simulink model "overall_simulator"  (R2018b)
settings: Solver=VariableStepAuto  StartTime=0.0  StopTime=100  RelTol=1e-3
InitFcn:
  | Iyy_lbft2= 261.096376; %last updated 7 Dec 2018
  | Iyy = 0.04214011 *Iyy_lbft2;
  | initial_conds
values from neighbouring files (symbols this model uses):
  desired_vel = 15    [initial_conds.m]
  flap_angle = 0    [initial_conds.m]
  initial_attitude = 0    [initial_conds.m]
  initial_incidence = 0    [initial_conds.m]
  motor_angle = 10    [initial_conds.m]
libraries: aerolibconvert2 x5, simulink x5, shared3dof x1, aerolibasang x1
settings Model: Creator=Devansh  LastModifiedBy=Alex
settings DebuggingCC: UnderSpecifiedDimensionMsg=warning
settings SFSimCC: SimUseLocalCustomCode=off
settings RTWCC: RTWUseLocalCustomCode=off
settings CodeAppCC: StateflowObjectComments=on

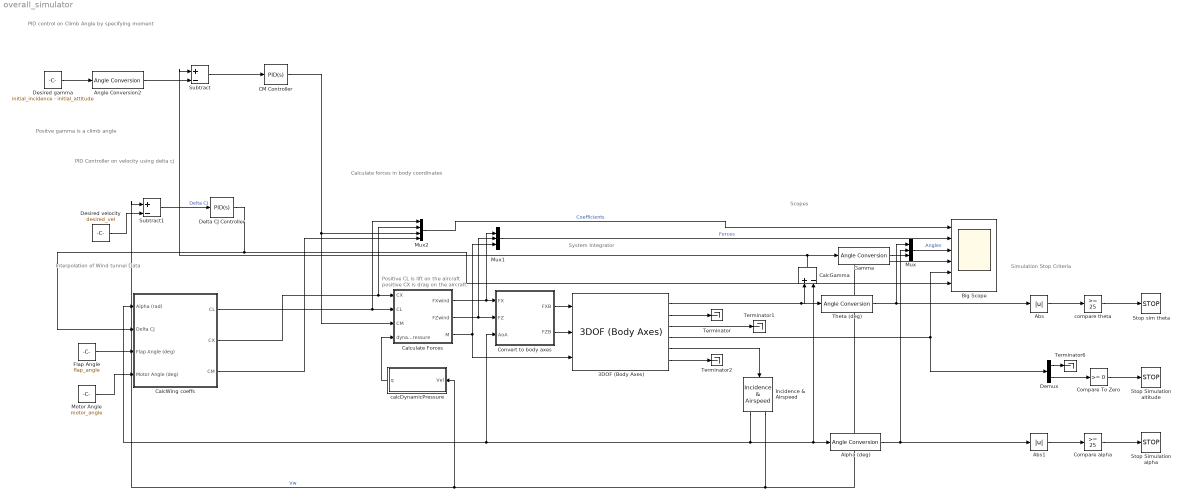
== system overall_simulator ==
  note: Positve gamma is a climb angle
  note: Scopes
  note: Simulation Stop Criteria
  note: System Integrator
  note: Calculate forces in body coordinates
  note: PID control on Climb Angle by specifying moment
  note: Interpolation of Wind tunnel Data
  note: PID Controller on velocity using delta cj
  note: Positive CL is lift on the aircraft
      | positive CX is drag on the aircraft
  3DOF (Body Axes) : shared3dof/3DOF (Body Axes)  units=Metric (MKS)  mtype=Fixed  v_ini=desired_vel  theta_ini=initial_attitude*pi/180  alpha_ini=initial_incidence*pi/180  pos_ini=initial_position  q_ini=0  mass=initial_mass  mass_e=0.5  mass_f=3.0  Iyy=Iyy  Iyy_e=0.5  Iyy_f=3.0  g_in=Internal  g=9.81  vre_flag=on  abi_flag=off  aMode=aMode  vel_statename=''  theta_statename=''  pos_statename=''  q_statename=''  mass_statename=''
      settings: SourceProductName=Aerospace Blockset  SourceProductBaseCode=AE
  Abs : Abs
  Abs1 : Abs
  Alpha (deg) : aerolibconvert2/Angle Conversion  IU=rad  OU=deg
  Angle Conversion2 : aerolibconvert2/Angle Conversion  IU=deg  OU=rad
  Big Scope : Scope  NumInputPorts=6
  CM Controller : simulink/Continuous/PID Controller  Controller=PID  Form=Parallel  TimeDomain=Continuous-time  SampleTime=-1  IntegratorMethod=Forward Euler  FilterMethod=Forward Euler  ControllerParametersSource=internal  P=-.005  I=0  D=-.05  UseFilter=on  N=100  TunerSelectOption=Frequency Response Based  InitialConditionSource=internal  InitialConditionForIntegrator=0  InitialConditionForFilter=0  DifferentiatorICPrevScaledInput=0  ExternalReset=none  TrackingMode=off  Kt=1  LimitOutput=off  UpperSaturationLimit=0.1  LowerSaturationLimit=-0.1  LinearizeAsGain=off  AntiWindupMode=none  Kb=1  POutMin=[]  POutMax=[]  IOutMin=[]  IOutMax=[]  DOutMin=[]  DOutMax=[]  NOutMin=[]  NOutMax=[]  SumOutMin=[]  SumOutMax=[]  SaturationOutMin=[]  SaturationOutMax=[]  PParamMin=[]  PParamMax=[]  IParamMin=[]  IParamMax=[]  DParamMin=[]  DParamMax=[]  NParamMin=[]  NParamMax=[]  KbParamMin=[]  KbParamMax=[]  KtParamMin=[]  KtParamMax=[]  KbOutMin=[]  KbOutMax=[]  KtOutMin=[]  KtOutMax=[]  IntegratorOutMin=[]  IntegratorOutMax=[]  FilterOutMin=[]  FilterOutMax=[]  SumI1OutMin=[]  SumI1OutMax=[]  SumI2OutMin=[]  SumI2OutMax=[]  SumI3OutMin=[]  SumI3OutMax=[]  SumI4OutMin=[]  SumI4OutMax=[]  SumDOutMin=[]  SumDOutMax=[]  DifferentiatorOutMin=[]  DifferentiatorOutMax=[]  FilterDiffOutCoefMin=[]  FilterDiffOutCoefMax=[]  ReciprocalOutMin=[]  ReciprocalOutMax=[]  SumDenOutMin=[]  SumDenOutMax=[]  SumNumOutMin=[]  SumNumOutMax=[]  DivideOutMin=[]  DivideOutMax=[]  IntegratorContinuousStateAttributes=''  IntegratorStateMustResolveToSignalObject=off  IntegratorRTWStateStorageClass=Auto  FilterContinuousStateAttributes=''  FilterStateMustResolveToSignalObject=off  FilterRTWStateStorageClass=Auto  ParallelPVariant=InternalParameters  IdealPVariant=Disabled  IVariant=InternalParameters  DVariant=InternalParameters  IntegratorVariant=Continuous  SatVariant=Disabled  AWVariant=Passthrough  PCopyVariant=Disabled  TRVariant=Disabled  FdbkBlocksVariant=Forward  IdealPFdbkVariant=Disabled  SatFdbkVariant=Disabled  DerivativeFilterVariant=ContFilter  NVariant=InternalParameters  NCopyVariant=Disabled  FilterICVariant=InternalICsFilter  IntegratorICVariant=InternalICs  ExternalResetVariant=Disabled  TRSumVariant=Passthrough  SumFdbkVariant=Disabled  SumVariant=Sum_PID
  CalcGamma : Sum  Inputs=+|-
  CalcWing coeffs : Subsystem
  Calculate Forces : Subsystem
  Compare To Zero : simulink/Logic and Bit Operations/Compare To Zero  relop=>=  OutDataTypeStr=boolean
  Compare alpha : simulink/Logic and Bit Operations/Compare To Constant  relop=>=  const=25  OutDataTypeStr=boolean
  Convert to body axes : Subsystem
  Delta CJ Controller : simulink/Continuous/PID Controller  Controller=PID  Form=Parallel  TimeDomain=Continuous-time  SampleTime=-1  IntegratorMethod=Forward Euler  FilterMethod=Forward Euler  ControllerParametersSource=internal  P=-0.5  I=-2  D=0  UseFilter=on  N=100  TunerSelectOption=Transfer Function Based (PID Tuner App)  InitialConditionSource=internal  InitialConditionForIntegrator=0  InitialConditionForFilter=0  DifferentiatorICPrevScaledInput=0  ExternalReset=none  TrackingMode=off  Kt=1  LimitOutput=on  UpperSaturationLimit=6  LowerSaturationLimit=0  LinearizeAsGain=off  AntiWindupMode=none  Kb=1  POutMin=[]  POutMax=[]  IOutMin=[]  IOutMax=[]  DOutMin=[]  DOutMax=[]  NOutMin=[]  NOutMax=[]  SumOutMin=[]  SumOutMax=[]  SaturationOutMin=[]  SaturationOutMax=[]  PParamMin=[]  PParamMax=[]  IParamMin=[]  IParamMax=[]  DParamMin=[]  DParamMax=[]  NParamMin=[]  NParamMax=[]  KbParamMin=[]  KbParamMax=[]  KtParamMin=[]  KtParamMax=[]  KbOutMin=[]  KbOutMax=[]  KtOutMin=[]  KtOutMax=[]  IntegratorOutMin=[]  IntegratorOutMax=[]  FilterOutMin=[]  FilterOutMax=[]  SumI1OutMin=[]  SumI1OutMax=[]  SumI2OutMin=[]  SumI2OutMax=[]  SumI3OutMin=[]  SumI3OutMax=[]  SumI4OutMin=[]  SumI4OutMax=[]  SumDOutMin=[]  SumDOutMax=[]  DifferentiatorOutMin=[]  DifferentiatorOutMax=[]  FilterDiffOutCoefMin=[]  FilterDiffOutCoefMax=[]  ReciprocalOutMin=[]  ReciprocalOutMax=[]  SumDenOutMin=[]  SumDenOutMax=[]  SumNumOutMin=[]  SumNumOutMax=[]  DivideOutMin=[]  DivideOutMax=[]  IntegratorContinuousStateAttributes=''  IntegratorStateMustResolveToSignalObject=off  IntegratorRTWStateStorageClass=Auto  FilterContinuousStateAttributes=''  FilterStateMustResolveToSignalObject=off  FilterRTWStateStorageClass=Auto  ParallelPVariant=InternalParameters  IdealPVariant=Disabled  IVariant=InternalParameters  DVariant=InternalParameters  IntegratorVariant=Continuous  SatVariant=Enabled  AWVariant=Passthrough  PCopyVariant=Disabled  TRVariant=Disabled  FdbkBlocksVariant=Forward  IdealPFdbkVariant=Disabled  SatFdbkVariant=Disabled  DerivativeFilterVariant=ContFilter  NVariant=InternalParameters  NCopyVariant=Disabled  FilterICVariant=InternalICsFilter  IntegratorICVariant=InternalICs  ExternalResetVariant=Disabled  TRSumVariant=Passthrough  SumFdbkVariant=Disabled  SumVariant=Sum_PID
  Demux : Demux  Outputs=2
  "Desired gamma " : Constant  Value=initial_incidence - initial_attitude
  Desired velocity : Constant  Value=desired_vel
  Flap Angle : Constant  Value=flap_angle
  Gamma : aerolibconvert2/Angle Conversion  IU=rad  OU=deg
  Incidence & Airspeed : aerolibasang/Incidence  & Airspeed
      settings: SourceProductName=Aerospace Blockset  SourceProductBaseCode=AE
  Motor Angle : Constant  Value=motor_angle
  Mux : Mux  Inputs=3
  Mux1 : Mux  Inputs=3
  Mux2 : Mux
  Stop Simulation alpha : Stop
  Stop Simulation altitude : Stop
  Stop sim theta : Stop
  Subtract : Sum  Inputs=+|-
  Subtract1 : Sum  Inputs=+|-
  Terminator{,1..2,6} (4 alike) : Terminator
  Theta (deg) : aerolibconvert2/Angle Conversion  IU=rad  OU=deg
  calcDynamicPressure : Subsystem  TreatAsAtomicUnit=on
  compare theta : simulink/Logic and Bit Operations/Compare To Constant  relop=>=  const=25  OutDataTypeStr=boolean
  wires:
  3DOF (Body Axes)/4 -> Big Scope/5, Demux/1
  Theta (deg)/1 -> Mux/1, Abs/1
  Alpha (deg)/1 -> Abs1/1, Mux/2
  Demux/2 -> Compare To Zero/1
  Compare To Zero/1 -> Stop Simulation altitude/1
  Incidence & Airspeed/2 -> Big Scope/4, Subtract1/1, calcDynamicPressure/1(Vel)  "Vw"
  "Desired gamma "/1 -> Angle Conversion2/1
  Angle Conversion2/1 -> Subtract/2
  CalcWing coeffs/1(CL) -> Mux2/1, Calculate Forces/2(CL)
  calcDynamicPressure/1(q) -> Calculate Forces/4(dynamicPressure)
  Calculate Forces/1(FXwind) -> Mux1/1, Convert to body axes/1(FX)
  Calculate Forces/2(FZwind) -> Mux1/2, Convert to body axes/2(FZ)
  Calculate Forces/3(M) -> Mux1/3, 3DOF (Body Axes)/3
  3DOF (Body Axes)/2 -> Terminator/1
  3DOF (Body Axes)/3 -> Terminator1/1
  3DOF (Body Axes)/6 -> Terminator2/1
  Flap Angle/1 -> CalcWing coeffs/3(Flap Angle (deg))
  CalcWing coeffs/2(CX) -> Calculate Forces/1(CX), Mux2/2
  Motor Angle/1 -> CalcWing coeffs/4(Motor Angle (deg))
  compare theta/1 -> Stop sim theta/1
  Abs/1 -> compare theta/1
  Abs1/1 -> Compare alpha/1
  Incidence & Airspeed/1 -> CalcWing coeffs/1(Alpha (rad)), Convert to body axes/3(AoA), CalcGamma/2, Alpha (deg)/1
  Compare alpha/1 -> Stop Simulation alpha/1
  CalcWing coeffs/3(CM) -> Mux2/4
  Demux/1 -> Terminator6/1
  Subtract1/1 -> Delta CJ Controller/1  "Delta CJ"
  Desired velocity/1 -> Subtract1/2
  Delta CJ Controller/1 -> CalcWing coeffs/2(Delta CJ), Big Scope/6
  3DOF (Body Axes)/5 -> Incidence & Airspeed/1
  Convert to body axes/1(FXB) -> 3DOF (Body Axes)/1
  Convert to body axes/2(FZB) -> 3DOF (Body Axes)/2
  3DOF (Body Axes)/1 -> CalcGamma/1, Theta (deg)/1
  CalcGamma/1 -> Subtract/1, Gamma/1
  Gamma/1 -> Mux/3
  Mux/1 -> Big Scope/3  "Angles"
  Mux1/1 -> Big Scope/2  "Forces"
  Mux2/1 -> Big Scope/1  "Coefficients"
  CM Controller/1 -> Mux2/3, Calculate Forces/3(CM)
  Subtract/1 -> CM Controller/1

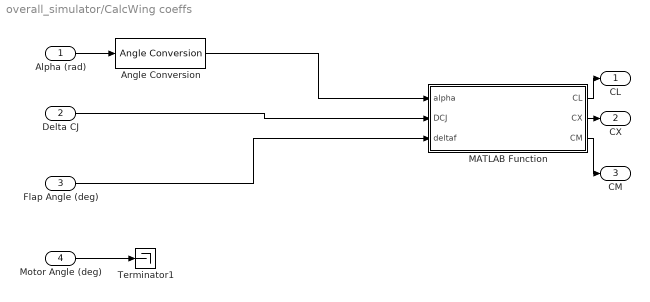
== system overall_simulator/CalcWing coeffs ==
  Alpha (rad) : Inport
  Delta CJ : Inport  Port=2
  Flap Angle (deg) : Inport  Port=3
  Motor Angle (deg) : Inport  Port=4
  Angle Conversion : aerolibconvert2/Angle Conversion  IU=rad  OU=deg
  MATLAB Function : MATLAB Function  TreatAsAtomicUnit=on
  Terminator1 : Terminator
  CL : Outport
  CX : Outport  Port=2
  CM : Outport  Port=3
  wires:
  Alpha (rad)/1 -> Angle Conversion/1
  Flap Angle (deg)/1 -> MATLAB Function/3(deltaf)
  Motor Angle (deg)/1 -> Terminator1/1
  MATLAB Function/1(CL) -> CL/1
  MATLAB Function/3(CM) -> CM/1
  MATLAB Function/2(CX) -> CX/1
  Angle Conversion/1 -> MATLAB Function/1(alpha)
  Delta CJ/1 -> MATLAB Function/2(DCJ)

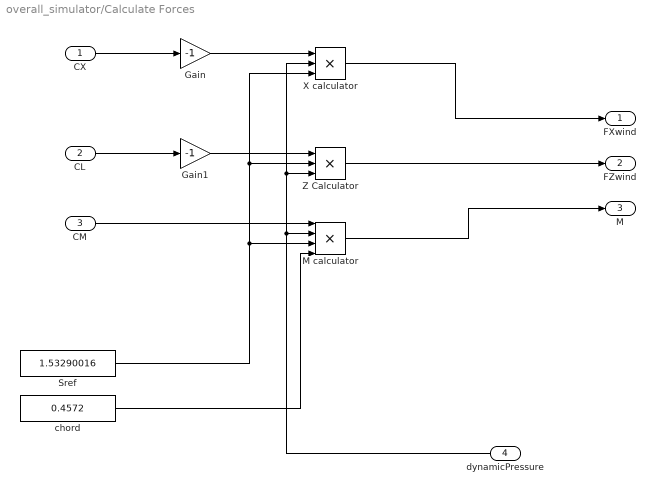
== system overall_simulator/Calculate Forces ==
  CX : Inport
  CL : Inport  Port=2
  CM : Inport  Port=3
  dynamicPressure : Inport  Port=4
  Gain : Gain  Gain=-1
  Gain1 : Gain  Gain=-1
  M calculator : Product  Inputs=4
  Sref : Constant  Value=1.53290016
  X calculator : Product  Inputs=3
  Z Calculator : Product  Inputs=3
  chord : Constant  Value=0.4572
  FXwind : Outport
  FZwind : Outport  Port=2
  M : Outport  Port=3
  wires:
  CM/1 -> M calculator/1
  M calculator/1 -> M/1
  chord/1 -> M calculator/4
  Sref/1 -> X calculator/3, Z Calculator/2, M calculator/3
  X calculator/1 -> FXwind/1
  dynamicPressure/1 -> X calculator/2, Z Calculator/3, M calculator/2
  Z Calculator/1 -> FZwind/1
  CX/1 -> Gain/1
  CL/1 -> Gain1/1
  Gain/1 -> X calculator/1
  Gain1/1 -> Z Calculator/1

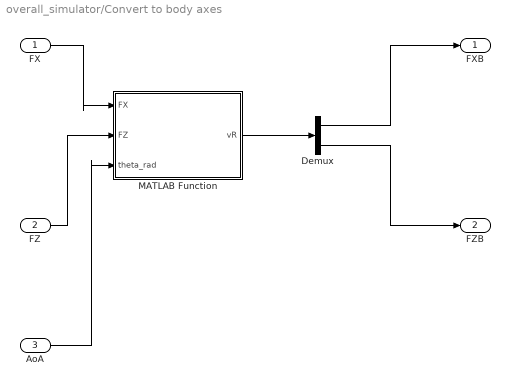
== system overall_simulator/Convert to body axes ==
  FX : Inport
  FZ : Inport  Port=2
  AoA : Inport  Port=3
  Demux : Demux  Outputs=2
  MATLAB Function : MATLAB Function  TreatAsAtomicUnit=on
  FXB : Outport
  FZB : Outport  Port=2
  wires:
  FX/1 -> MATLAB Function/1(FX)
  FZ/1 -> MATLAB Function/2(FZ)
  AoA/1 -> MATLAB Function/3(theta_rad)
  MATLAB Function/1(vR) -> Demux/1
  Demux/1 -> FXB/1
  Demux/2 -> FZB/1

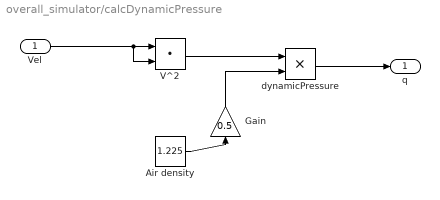
== system overall_simulator/calcDynamicPressure ==
  Vel : Inport
  Air density : Constant  Value=1.225
  Gain : Gain  Gain=0.5
  V^2 : DotProduct  InputSameDT=on  OutDataTypeStr=Inherit: Inherit via internal rule
  dynamicPressure : Product
  q : Outport
  wires:
  V^2/1 -> dynamicPressure/1
  Air density/1 -> Gain/1
  Vel/1 -> V^2/2, V^2/1
  dynamicPressure/1 -> q/1
  Gain/1 -> dynamicPressure/2

== matlab function overall_simulator/Convert to body axes/MATLAB Function ==
  data: FX input; vR output; FZ input; theta_rad input
function vR = rotation(FX, FZ, theta_rad)

v = [FX; FZ];

 R = [cos(theta_rad) -sin(theta_rad); sin(theta_rad) cos(theta_rad)];
 
 vR = R*v;

== matlab function overall_simulator/CalcWing coeffs/MATLAB Function ==
  data: alpha input; CL output; DCJ input; CX output; CM output; deltaf input
function [CL,CX,CM] = getCLCXCM_for_df40(alpha, DCJ, deltaf)

%% convert 3D Delta CJ to 2D

delta_cj=DCJ/0.85;

%% get coefficient matrix
%assumes delta f = 40;
if deltaf == 0
    CL_coeffs =[0.217960258381776 0.109138353113665 -0.000041729685398 0 0; -0.057543207773095 0.038658000373704 -0.000004063818321 0 0];

    CD_coeffs =[0.298029538315143 -0.032494869214750 0.001607648897644 0 0; -1.169404424397114 0.010531734054736 0.000383579742027 0 0];

    CM_coeffs = [-0.025987417994104 -0.003425926814426 -0.000000214240384 0 0; 0.047889195368891 0.000520651340568 0.000002162356444 0 0];
elseif deltaf == 20
    CL_coeffs =[0.470361634556928 0.149578298813986 -0.000207701035812 0 0; 0.364072012597468 0.039136516232660 0.000007889310247 0 0];

    CD_coeffs =[0.298024007875823 -0.077292745254834 0.004127544479797 0 0; -0.965158154402554 0.035738748181709 -0.000492093552988 0 0];

    CM_coeffs = [-0.061421743922260 -0.005202157247354 0.000004966549384 0 0; -0.039743527273597 0.001729293722182 0.000002768098075 0 0];
elseif deltaf == 40
    CL_coeffs =[1.34084802984238,0.0922989525732600,-0.000100934251419516,0,0;...
        0.840192956938716,0.0440183793695609,-2.84422877175519e-05,0,0];

    CD_coeffs =[0.217559985374938,-0.0212488590862297,0.00119201327474585,0,0;...
        -0.717426345875555,0.0291623276576992,-9.19585265352026e-05,0,0];

    CM_coeffs = [-0.209467748915995,0.000759426537477041,-1.11246051270488e-06,0,0;...
        -0.0980528447065869,-0.000645846214599032,7.76293222113931e-06,0,0];
else
    deltaf = 55;
    CL_coeffs =[1.168919251646413 0.089122576268785 -0.000289430618341 0 0; 0.558544900304277 0.023165937398060 0.000014806582549 0 0];

    CD_coeffs =[0.342006471367090 0.004773850866101 -0.000516749906378 0 0; -0.458718605607410 0.009102396612331 0.000202012706694 0 0];

    CM_coeffs = [-0.160407251082783 0.000219375516177 0.000010480723794 0 0; -0.077402435687801 0.000555520205222 0.000003121604777 0 0];
end

%% get regression results

%get cl
X=[];
for i=0:size(CL_coeffs,1)-1
    X=[X (delta_cj.^i)];
end

cl=X*CL_coeffs(:,1)+alpha.*(X*CL_coeffs(:,2))+alpha.^3.*(X*CL_coeffs(:,3))+deltaf.*(X*CL_coeffs(:,4))+deltaf.^3.*(X*CL_coeffs(:,5));

%get cx
X=[];
for i=0:size(CD_coeffs,1)-1
    X=[X (delta_cj.^i)];
end
cx=X*CD_coeffs(:,1)+alpha.*(X*CD_coeffs(:,2))+alpha.^2.*(X*CD_coeffs(:,3))+deltaf.*(X*CD_coeffs(:,4))+deltaf.^2.*(X*CD_coeffs(:,5));

%get cm
X=[];
for i=0:size(CM_coeffs,1)-1
    X=[X (delta_cj.^i)];
end
cm=X*CM_coeffs(:,1)+alpha.*(X*CM_coeffs(:,2))+alpha.^3.*(X*CM_coeffs(:,3))+deltaf.*(X*CM_coeffs(:,4))+deltaf.^3.*(X*CM_coeffs(:,5));


%% convert to 3D params
AR = 7.5;

e=0.9;
CT=DCJ-1;
CDp=0.05; %profile drag of the rest of the aircraft

CL=0.9*cl;
CX=0.9*cx+CDp+CL.^2./(pi*AR*e+2*CT);
CM = cm;


end
